simulink model "DealPosLrnd"  (R2018b)
settings: Solver=FixedStepDiscrete  StartTime=0.0  StopTime=10.0  FixedStep=0.01  RelTol=1e-3
undefined symbols (not defined in the file or in its folder): IfKeSMSbSeatMovBkRclnEnable_Val, IfKeSMSbSeatMovBlstOtwdInwdEnable_Val, IfKeSMSbSeatMovCshnFldEnable_Val, IfKeSMSbSeatMovCushnFrtEnable_Val, IfKeSMSbSeatMovFrwdBkwdEnable_Val, IfKeSMSbSeatMovFtrstEnable_Val, IfKeSMSbSeatMovLgrstEnable_Val, IfKeSMSbSeatMovLtwdRtwdEnable_Val, IfVeSMSeStNumConfig, KeSMSbArmscreenMovEnable_Val, KeSMSbIgnorePosLrnd_Val, KeSMSbSeatMovHdFrwdBkwdEnable_Val, KeSMSbSeatMovHdUpwdDnwdEnable_Val, KeSMSbSeatMovLgrstExpdEnable_Val
(part 1 of 2)
settings Model: Creator=su3dcu  LastModifiedBy=su3dcu
settings DataIOCC: SaveFormat=StructureWithTime  ReturnWorkspaceOutputs=on
settings OptimizationCC: DefaultParameterBehavior=Inlined  EnhancedBackFolding=on  PassReuseOutputArgsAs=Individual arguments  ZeroExternalMemoryAtStartup=off  ZeroInternalMemoryAtStartup=off  OptimizeBlockOrder=speed  DifferentSizesBufferReuse=on  OptimizationCustomize=off
settings DebuggingCC: ParameterTunabilityLossMsg=error
settings HardwareCC: ProdBitPerPointer=32  ProdBitPerSizeT=32  ProdBitPerPtrDiffT=32  ProdLargestAtomicFloat=None  ProdWordSize=32  ProdHWDeviceType=Renesas->RH850
settings ModelReferenceCC: ModelReferenceNumInstancesAllowed=Single
settings SFSimCC: SimCustomHeaderCode="#include\"Rte_Type.h\""  MATLABDynamicMemAlloc=off
settings RTWCC: SystemTargetFile=autosar.tlc  GenCodeOnly=on  TemplateMakefile=ert_default_tmf  Description=AUTOSAR  GenerateReport=on  IncludeHyperlinkInReport=on  LaunchReport=on  CodeExecutionProfiling=on  GenerateTraceInfo=on  GenerateTraceReport=on  GenerateTraceReportSl=on  GenerateTraceReportSf=on  GenerateTraceReportEml=on  GenerateCodeMetricsReport=on
settings CodeAppCC: ForceParamTrailComments=on  IgnoreCustomStorageClasses=off  MaxIdLength=63  OperatorAnnotations=on  SimulinkDataObjDesc=on  SFDataObjDesc=on  InsertBlockDesc=on
settings STFCustomTargetCC: TargetLangStandard=C99 (ISO)  MultiwordLength=256  ParMdlRefBuildCompliant=on  CompOptLevelCompliant=on  IncludeMdlTerminateFcn=off  CombineOutputUpdateFcns=on  SuppressErrorStatus=on  ERTCustomFileBanners=on  SupportAbsoluteTime=off  PurelyIntegerCode=on  SupportNonFinite=off  SupportComplex=off  SupportContinuousTime=off  SupportNonInlinedSFcns=off  RemoveResetFunc=on  MATLABClassNameForMDSCustomization=Simulink.SoftwareTarget.ERTCustomization  AutosarCompliant=on  UseToolchainInfoCompliant=on  LookupTableObjectStructAxisOrder=2,1,3,4,...  LUTObjectStructOrderEvenSpacing=Size,Table,Breakpoints  SystemTargetFile=autosar.tlc
settings ERTTargetCC: TargetLangStandard=C99 (ISO)  ConcurrentExecutionCompliant=off  IncludeMdlTerminateFcn=off  SuppressErrorStatus=on  SupportAbsoluteTime=off  PurelyIntegerCode=on  SupportNonFinite=off  SupportComplex=off  ModelStepFunctionPrototypeControlCompliant=off  CPPClassGenCompliant=off  AutosarCompliant=on  LookupTableObjectStructAxisOrder=2,1,3,4,...  LUTObjectStructOrderEvenSpacing=Size,Table,Breakpoints  InlinedParameterPlacement=NonHierarchical  ERTCustomFileTemplate=example_file_process.tlc  ERTFilePackagingFormat=Compact
settings ConfigComp: DVTestSuiteOptimization=CombinedObjectives (Nonlinear Extended)  DVDetectActiveLogic=on  DVDetectOutOfBounds=on

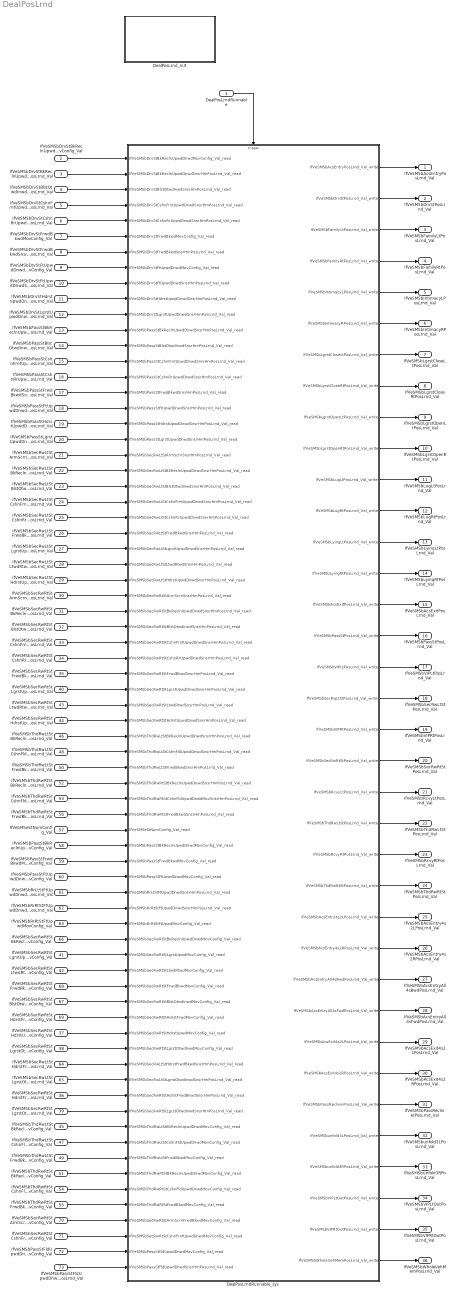
== system DealPosLrnd ==
  DealPosLrndRunnable : Inport  SampleTime=0.01  OutputFunctionCall=on
  IfVeSMSbDrvStBkReclnUpwdDnwdMovConfig_Val : Inport  Port=2  OutDataTypeStr=boolean  PortDimensions=1
  IfVeSMSbDrvStBkReclnUpwdDnwdSnsrHmPosLrnd_Val : Inport  Port=3  OutDataTypeStr=PosLrnd1  PortDimensions=1
  IfVeSMSbDrvStBlstOtwdInwdSnsrHmPosLrnd_Val : Inport  Port=4  OutDataTypeStr=PosLrnd1  PortDimensions=1
  IfVeSMSbDrvStCshnFrntUpwdDnwdSnsrHmPosLrnd_Val : Inport  Port=5  OutDataTypeStr=PosLrnd1  PortDimensions=1
  IfVeSMSbDrvStCshnRrUpwdDnwdSnsrHmPosLrnd_Val : Inport  Port=6  OutDataTypeStr=PosLrnd1  PortDimensions=1
  IfVeSMSbDrvStFrwdBkwdMovConfig_Val : Inport  Port=7  OutDataTypeStr=boolean  PortDimensions=1
  IfVeSMSbDrvStFrwdBkwdSnsrHmPosLrnd_Val : Inport  Port=8  OutDataTypeStr=PosLrnd1  PortDimensions=1
  IfVeSMSbDrvStFtUpwdDnwdMovConfig_Val : Inport  Port=9  OutDataTypeStr=boolean  PortDimensions=1
  IfVeSMSbDrvStFtUpwdDnwdSnsrHmPosLrnd_Val : Inport  Port=10  OutDataTypeStr=PosLrnd1  PortDimensions=1
  IfVeSMSbDrvStHdrstUpwdDnwdSnsrHmPosLrnd_Val : Inport  Port=11  OutDataTypeStr=PosLrnd1  PortDimensions=1
  IfVeSMSbDrvStLgrstUpwdDnwdSnsrHmPosLrnd_Val : Inport  Port=12  OutDataTypeStr=PosLrnd1  PortDimensions=1
  IfVeSMSbPassStBkReclnUpwdDnwdSnsrHmPosLrnd_Val : Inport  Port=13  OutDataTypeStr=PosLrnd1  PortDimensions=1
  IfVeSMSbPassStBlstOtwdInwdSnsrHmPosLrnd_Val : Inport  Port=14  OutDataTypeStr=PosLrnd1  PortDimensions=1
  IfVeSMSbPassStCshnFrntUpwdDnwdSnsrHmPosLrnd_Val : Inport  Port=15  OutDataTypeStr=PosLrnd1  PortDimensions=1
  IfVeSMSbPassStCshnRrUpwdDnwdSnsrHmPosLrnd_Val : Inport  Port=16  OutDataTypeStr=PosLrnd1  PortDimensions=1
  IfVeSMSbPassStFrwdBkwdSnsrHmPosLrnd_Val : Inport  Port=17  OutDataTypeStr=PosLrnd1  PortDimensions=1
  IfVeSMSbPassStFtUpwdDnwdSnsrHmPosLrnd_Val : Inport  Port=18  OutDataTypeStr=PosLrnd1  PortDimensions=1
  IfVeSMSbPassStHdrstUpwdDnwdSnsrHmPosLrnd_Val : Inport  Port=19  OutDataTypeStr=PosLrnd1  PortDimensions=1
  IfVeSMSbPassStLgrstUpwdDnwdSnsrHmPosLrnd_Val : Inport  Port=20  OutDataTypeStr=PosLrnd1  PortDimensions=1
  IfVeSMSbSecRwLtStArmScrnSnsrHmPosLrnd_Val : Inport  Port=21  OutDataTypeStr=PosLrnd1  PortDimensions=1
  IfVeSMSbSecRwLtStBkReclnUpwdDnwdSnsrHmPosLrnd_Val : Inport  Port=22  OutDataTypeStr=PosLrnd1  PortDimensions=1
  IfVeSMSbSecRwLtStBlstOtwdInwdSnsrHmPosLrnd_Val : Inport  Port=23  OutDataTypeStr=PosLrnd1  PortDimensions=1
  IfVeSMSbSecRwLtStCshnFrntUpwdDnwdSnsrHmPosLrnd_Val : Inport  Port=24  OutDataTypeStr=PosLrnd1  PortDimensions=1
  IfVeSMSbSecRwLtStCshnRrUpwdDnwdSnsrHmPosLrnd_Val : Inport  Port=25  OutDataTypeStr=PosLrnd1  PortDimensions=1
  IfVeSMSbSecRwLtStFrwdBkwdSnsrHmPosLrnd_Val : Inport  Port=26  OutDataTypeStr=PosLrnd1  PortDimensions=1
  IfVeSMSbSecRwLtStLgrstUpwdDnwdSnsrHmPosLrnd_Val : Inport  Port=27  OutDataTypeStr=PosLrnd1  PortDimensions=1
  IfVeSMSbSecRwLtStLtwdRtwdSnsrHmPosLrnd_Val : Inport  Port=28  OutDataTypeStr=PosLrnd1  PortDimensions=1
  IfVeSMSbSecRwLtStHdrstUpwdDnwdSnsrHmPosLrnd_Val : Inport  Port=29  OutDataTypeStr=PosLrnd1  PortDimensions=1
  IfVeSMSbSecRwRtStArmScrnSnsrHmPosLrnd_Val : Inport  Port=30  OutDataTypeStr=PosLrnd1  PortDimensions=1
  IfVeSMSbSecRwRtStBkReclnUpwdDnwdSnsrHmPosLrnd_Val : Inport  Port=31  OutDataTypeStr=PosLrnd1  PortDimensions=1
  IfVeSMSbSecRwRtStBlstOtwdInwdSnsrHmPosLrnd_Val : Inport  Port=32  OutDataTypeStr=PosLrnd1  PortDimensions=1
  IfVeSMSbSecRwRtStCshnFrntUpwdDnwdSnsrHmPosLrnd_Val : Inport  Port=33  OutDataTypeStr=PosLrnd1  PortDimensions=1
  IfVeSMSbSecRwRtStCshnRrUpwdDnwdSnsrHmPosLrnd_Val : Inport  Port=34  OutDataTypeStr=PosLrnd1  PortDimensions=1
  IfVeSMSbSecRwRtStFrwdBkwdSnsrHmPosLrnd_Val : Inport  Port=35  OutDataTypeStr=PosLrnd1  PortDimensions=1
  IfVeSMSbSecRwRtStHdrstFrwdBkwdSnsrHmPosLrnd_Val : Inport  Port=36  OutDataTypeStr=PosLrnd1  PortDimensions=1
  IfVeSMSbSecRwRtStHdrstUpwdMovConfig_Val : Inport  Port=37  OutDataTypeStr=boolean  PortDimensions=1
  IfVeSMSbSecRwRtStLgrstOtwdInwdMovConfig_Val : Inport  Port=38  OutDataTypeStr=boolean  PortDimensions=1
  IfVeSMSbSecRwRtStLgrstOtwdInwdSnsrHmPosLrnd_Val : Inport  Port=39  OutDataTypeStr=PosLrnd1  PortDimensions=1
  IfVeSMSbSecRwRtStLgrstUpwdDnwdSnsrHmPosLrnd_Val : Inport  Port=40  OutDataTypeStr=PosLrnd1  PortDimensions=1
  IfVeSMSbSecRwRtStLgrstUpwdMovConfig_Val : Inport  Port=41  OutDataTypeStr=boolean  PortDimensions=1
  IfVeSMSbSecRwRtStLtwdRtwdMovConfig_Val : Inport  Port=42  OutDataTypeStr=boolean  PortDimensions=1
  IfVeSMSbSecRwRtStLtwdRtwdSnsrHmPosLrnd_Val : Inport  Port=43  OutDataTypeStr=PosLrnd1  PortDimensions=1
  IfVeSMSbSecRwRtStHdrstUpwdDnwdSnsrHmPosLrnd_Val : Inport  Port=44  OutDataTypeStr=PosLrnd1  PortDimensions=1
  IfVeSMSbThdRwLtStBkReclnUpwdDnwdMovConfig_Val : Inport  Port=45  OutDataTypeStr=boolean  PortDimensions=1
  IfVeSMSbThdRwLtStBkReclnUpwdDnwdSnsrHmPosLrnd_Val : Inport  Port=46  OutDataTypeStr=PosLrnd1  PortDimensions=1
  IfVeSMSbThdRwLtStCshnFldUpwdDnwdMovConfig_Val : Inport  Port=47  OutDataTypeStr=boolean  PortDimensions=1
  IfVeSMSbThdRwLtStCshnFldUpwdDnwdSnsrHmPosLrnd_Val : Inport  Port=48  OutDataTypeStr=PosLrnd1  PortDimensions=1
  IfVeSMSbThdRwLtStFrwdBkwdMovConfig_Val : Inport  Port=49  OutDataTypeStr=boolean  PortDimensions=1
  IfVeSMSbThdRwLtStFrwdBkwdSnsrHmPosLrnd_Val : Inport  Port=50  OutDataTypeStr=PosLrnd1  PortDimensions=1
  IfVeSMSbThdRwRtStBkReclnUpwdDnwdMovConfig_Val : Inport  Port=51  OutDataTypeStr=boolean  PortDimensions=1
  IfVeSMSbThdRwRtStBkReclnUpwdDnwdSnsrHmPosLrnd_Val : Inport  Port=52  OutDataTypeStr=PosLrnd1  PortDimensions=1
  IfVeSMSbThdRwRtStCshnFldUpwdDnwdMovSnsrHmPosLrnd_Val : Inport  Port=53  OutDataTypeStr=PosLrnd1  PortDimensions=1
  IfVeSMSbThdRwRtStCshnFldUpwdDnwdMovConfig_Val : Inport  Port=54  OutDataTypeStr=boolean  PortDimensions=1
  IfVeSMSbThdRwRtStFrwdBkwdMovConfig_Val : Inport  Port=55  OutDataTypeStr=boolean  PortDimensions=1
  IfVeSMSbThdRwRtStFrwdBkwdSnsrHmPosLrnd_Val : Inport  Port=56  OutDataTypeStr=PosLrnd1  PortDimensions=1
  IfVeSMSeStNumConfig_Val : Inport  Port=57  OutDataTypeStr=Enum: IfVeSMSeStNumConfig  PortDimensions=1
  IfVeSMSbPassStBkReclnUpwdDnwdMovConfig_Val : Inport  Port=58  OutDataTypeStr=boolean  PortDimensions=1
  IfVeSMSbPassStFrwdBkwdMovConfig_Val : Inport  Port=59  OutDataTypeStr=boolean  PortDimensions=1
  IfVeSMSbPassStFtUpwdDnwdMovConfig_Val : Inport  Port=60  OutDataTypeStr=boolean  PortDimensions=1
  IfVeSMSbRrLtStFtUpwdDnwdSnsrHmPosLrnd_Val : Inport  Port=61  OutDataTypeStr=PosLrnd1  PortDimensions=1
  IfVeSMSbRrRtStFtUpwdDnwdSnsrHmPosLrnd_Val : Inport  Port=62  OutDataTypeStr=PosLrnd1  PortDimensions=1
  IfVeSMSbRrRtStFtUpwdMovConfig_Val : Inport  Port=63  OutDataTypeStr=boolean  PortDimensions=1
  IfVeSMSbSecRwLtStHdrstFrwdBkwdSnsrHmPosLrnd_Val : Inport  Port=64  OutDataTypeStr=PosLrnd1  PortDimensions=1
  IfVeSMSbSecRwLtStLgrstOtwdInwdSnsrHmPosLrnd_Val : Inport  Port=65  OutDataTypeStr=PosLrnd1  PortDimensions=1
  IfVeSMSbSecRwRtStBkReclnUpwdDnwdMovConfig_Val : Inport  Port=66  OutDataTypeStr=boolean  PortDimensions=1
  IfVeSMSbSecRwRtStBlstOtwdInwdMovConfig_Val : Inport  Port=67  OutDataTypeStr=boolean  PortDimensions=1
  IfVeSMSbSecRwRtStFrwdBkwdMovConfig_Val : Inport  Port=68  OutDataTypeStr=boolean  PortDimensions=1
  IfVeSMSbSecRwRtStHdrstFrwdMovConfig_Val : Inport  Port=69  OutDataTypeStr=boolean  PortDimensions=1
  IfVeSMSbSecRwRtStArmScrnFrwdBkwdMovConfig_Val : Inport  Port=70  OutDataTypeStr=boolean  PortDimensions=1
  IfVeSMSbSecRwRtStCshnFrntUpwdDnwdMovConfig_Val : Inport  Port=71  OutDataTypeStr=boolean  PortDimensions=1
  IfVeSMSbPassStFldUpwdDnwdMovConfig_Val : Inport  Port=72  OutDataTypeStr=boolean  PortDimensions=1
  IfVeSMSbPassStFldUpwdDnwdSnsrHmPosLrnd_Val : Inport  Port=73  OutDataTypeStr=PosLrnd1  PortDimensions=1
  DealPosLrndRunnable_sys : Subsystem
  DealPosLrnd_Init : Subsystem
  IfVeSMSbAcsEntryPosLrnd_Val : Outport  OutDataTypeStr=PosLrnd1  PortDimensions=1
  IfVeSMSbDrvStPosLrnd_Val : Outport  Port=2  OutDataTypeStr=PosLrnd1  PortDimensions=1
  IfVeSMSbFamilyLtPosLrnd_Val : Outport  Port=3  OutDataTypeStr=PosLrnd1  PortDimensions=1
  IfVeSMSbFamilyRtPosLrnd_Val : Outport  Port=4  OutDataTypeStr=PosLrnd1  PortDimensions=1
  IfVeSMSbIntimacyLPosLrnd_Val : Outport  Port=5  OutDataTypeStr=PosLrnd1  PortDimensions=1
  IfVeSMSbIntimacyRPosLrnd_Val : Outport  Port=6  OutDataTypeStr=PosLrnd1  PortDimensions=1
  IfVeSMSbLgrstCloseLtPosLrnd_Val : Outport  Port=7  OutDataTypeStr=PosLrnd1  PortDimensions=1
  IfVeSMSbLgrstCloseRtPosLrnd_Val : Outport  Port=8  OutDataTypeStr=PosLrnd1  PortDimensions=1
  IfVeSMSbLgrstOpenLtPosLrnd_Val : Outport  Port=9  OutDataTypeStr=PosLrnd1  PortDimensions=1
  IfVeSMSbLgrstOpenRtPosLrnd_Val : Outport  Port=10  OutDataTypeStr=PosLrnd1  PortDimensions=1
  IfVeSMSbLugLtPosLrnd_Val : Outport  Port=11  OutDataTypeStr=PosLrnd1  PortDimensions=1
  IfVeSMSbLugRtPosLrnd_Val : Outport  Port=12  OutDataTypeStr=PosLrnd1  PortDimensions=1
  IfVeSMSbLyingLtPosLrnd_Val : Outport  Port=13  OutDataTypeStr=PosLrnd1  PortDimensions=1
  IfVeSMSbLyingRtPosLrnd_Val : Outport  Port=14  OutDataTypeStr=PosLrnd1  PortDimensions=1
  IfVeSMSbAcsExitPosLrnd_Val : Outport  Port=15  OutDataTypeStr=PosLrnd1  PortDimensions=1
  IfVeSMSbPassStPosLrnd_Val : Outport  Port=16  OutDataTypeStr=PosLrnd1  PortDimensions=1
  IfVeSMSbVIPLtPosLrnd_Val : Outport  Port=17  OutDataTypeStr=PosLrnd1  PortDimensions=1
  IfVeSMSbSecRwLtStPosLrnd_Val : Outport  Port=18  OutDataTypeStr=PosLrnd1  PortDimensions=1
  IfVeSMSbVIPRtPosLrnd_Val : Outport  Port=19  OutDataTypeStr=PosLrnd1  PortDimensions=1
  IfVeSMSbSecRwRtStPosLrnd_Val : Outport  Port=20  OutDataTypeStr=PosLrnd1  PortDimensions=1
  IfVeSMSbRcvyLtPosLrnd_Val : Outport  Port=21  OutDataTypeStr=PosLrnd1  PortDimensions=1
  IfVeSMSbThdRwLtStPosLrnd_Val : Outport  Port=22  OutDataTypeStr=PosLrnd1  PortDimensions=1
  IfVeSMSbRcvyRtPosLrnd_Val : Outport  Port=23  OutDataTypeStr=PosLrnd1  PortDimensions=1
  IfVeSMSbThdRwRtStPosLrnd_Val : Outport  Port=24  OutDataTypeStr=PosLrnd1  PortDimensions=1
  IfVeSMSbAcsEntry4s2LPosLrnd_Val : Outport  Port=25  OutDataTypeStr=PosLrnd1  PortDimensions=1
  IfVeSMSbAcsEntry4s2RPosLrnd_Val : Outport  Port=26  OutDataTypeStr=PosLrnd1  PortDimensions=1
  IfVeSMSbAcsEntryAll4sBwdPosLrnd_Val : Outport  Port=27  OutDataTypeStr=PosLrnd1  PortDimensions=1
  IfVeSMSbAcsEntryAll4sFwdPosLrnd_Val : Outport  Port=28  OutDataTypeStr=PosLrnd1  PortDimensions=1
  IfVeSMSbAcsExit4s2LPosLrnd_Val : Outport  Port=29  OutDataTypeStr=PosLrnd1  PortDimensions=1
  IfVeSMSbAcsExit4s2RPosLrnd_Val : Outport  Port=30  OutDataTypeStr=PosLrnd1  PortDimensions=1
  IfVeSMSbPassReclinerPosLrnd_Val : Outport  Port=31  OutDataTypeStr=PosLrnd1  PortDimensions=1
  IfVeSMSbunfold3LPosLrnd_Val : Outport  Port=32  OutDataTypeStr=PosLrnd1  PortDimensions=1
  IfVeSMSbunfold3RPosLrnd_Val : Outport  Port=33  OutDataTypeStr=PosLrnd1  PortDimensions=1
  IfVeSMSbVIPLtOutPosLrnd_Val : Outport  Port=34  OutDataTypeStr=PosLrnd1  PortDimensions=1
  IfVeSMSbVIPRtOutPosLrnd_Val : Outport  Port=35  OutDataTypeStr=PosLrnd1  PortDimensions=1
  IfVeSMSbWholeVehMemPosLrnd_Val : Outport  Port=36  OutDataTypeStr=PosLrnd1  PortDimensions=1
  wires:
  IfVeSMSbDrvStBkReclnUpwdDnwdMovConfig_Val/1 -> DealPosLrndRunnable_sys/1(IfVeSMSbDrvStBkReclnUpwdDnwdMovConfig_Val_read)
  IfVeSMSbDrvStBkReclnUpwdDnwdSnsrHmPosLrnd_Val/1 -> DealPosLrndRunnable_sys/2(IfVeSMSbDrvStBkReclnUpwdDnwdSnsrHmPosLrnd_Val_read)
  IfVeSMSbDrvStBlstOtwdInwdSnsrHmPosLrnd_Val/1 -> DealPosLrndRunnable_sys/3(IfVeSMSbDrvStBlstOtwdInwdSnsrHmPosLrnd_Val_read)
  IfVeSMSbDrvStCshnFrntUpwdDnwdSnsrHmPosLrnd_Val/1 -> DealPosLrndRunnable_sys/4(IfVeSMSbDrvStCshnFrntUpwdDnwdSnsrHmPosLrnd_Val_read)
  IfVeSMSbDrvStCshnRrUpwdDnwdSnsrHmPosLrnd_Val/1 -> DealPosLrndRunnable_sys/5(IfVeSMSbDrvStCshnRrUpwdDnwdSnsrHmPosLrnd_Val_read)
  IfVeSMSbDrvStFrwdBkwdMovConfig_Val/1 -> DealPosLrndRunnable_sys/6(IfVeSMSbDrvStFrwdBkwdMovConfig_Val_read)
  IfVeSMSbDrvStFrwdBkwdSnsrHmPosLrnd_Val/1 -> DealPosLrndRunnable_sys/7(IfVeSMSbDrvStFrwdBkwdSnsrHmPosLrnd_Val_read)
  IfVeSMSbDrvStFtUpwdDnwdMovConfig_Val/1 -> DealPosLrndRunnable_sys/8(IfVeSMSbDrvStFtUpwdDnwdMovConfig_Val_read)
  IfVeSMSbDrvStFtUpwdDnwdSnsrHmPosLrnd_Val/1 -> DealPosLrndRunnable_sys/9(IfVeSMSbDrvStFtUpwdDnwdSnsrHmPosLrnd_Val_read)
  IfVeSMSbDrvStHdrstUpwdDnwdSnsrHmPosLrnd_Val/1 -> DealPosLrndRunnable_sys/10(IfVeSMSbDrvStHdrstUpwdDnwdSnsrHmPosLrnd_Val_read)
  IfVeSMSbDrvStLgrstUpwdDnwdSnsrHmPosLrnd_Val/1 -> DealPosLrndRunnable_sys/11(IfVeSMSbDrvStLgrstUpwdDnwdSnsrHmPosLrnd_Val_read)
  IfVeSMSbPassStBkReclnUpwdDnwdSnsrHmPosLrnd_Val/1 -> DealPosLrndRunnable_sys/12(IfVeSMSbPassStBkReclnUpwdDnwdSnsrHmPosLrnd_Val_read)
  IfVeSMSbPassStBlstOtwdInwdSnsrHmPosLrnd_Val/1 -> DealPosLrndRunnable_sys/13(IfVeSMSbPassStBlstOtwdInwdSnsrHmPosLrnd_Val_read)
  IfVeSMSbPassStCshnFrntUpwdDnwdSnsrHmPosLrnd_Val/1 -> DealPosLrndRunnable_sys/14(IfVeSMSbPassStCshnFrntUpwdDnwdSnsrHmPosLrnd_Val_read)
  IfVeSMSbPassStCshnRrUpwdDnwdSnsrHmPosLrnd_Val/1 -> DealPosLrndRunnable_sys/15(IfVeSMSbPassStCshnRrUpwdDnwdSnsrHmPosLrnd_Val_read)
  IfVeSMSbPassStFrwdBkwdSnsrHmPosLrnd_Val/1 -> DealPosLrndRunnable_sys/16(IfVeSMSbPassStFrwdBkwdSnsrHmPosLrnd_Val_read)
  IfVeSMSbPassStFtUpwdDnwdSnsrHmPosLrnd_Val/1 -> DealPosLrndRunnable_sys/17(IfVeSMSbPassStFtUpwdDnwdSnsrHmPosLrnd_Val_read)
  IfVeSMSbPassStHdrstUpwdDnwdSnsrHmPosLrnd_Val/1 -> DealPosLrndRunnable_sys/18(IfVeSMSbPassStHdrstUpwdDnwdSnsrHmPosLrnd_Val_read)
  IfVeSMSbPassStLgrstUpwdDnwdSnsrHmPosLrnd_Val/1 -> DealPosLrndRunnable_sys/19(IfVeSMSbPassStLgrstUpwdDnwdSnsrHmPosLrnd_Val_read)
  IfVeSMSbSecRwLtStArmScrnSnsrHmPosLrnd_Val/1 -> DealPosLrndRunnable_sys/20(IfVeSMSbSecRwLtStArmScrnSnsrHmPosLrnd_Val_read)
  IfVeSMSbSecRwLtStBkReclnUpwdDnwdSnsrHmPosLrnd_Val/1 -> DealPosLrndRunnable_sys/21(IfVeSMSbSecRwLtStBkReclnUpwdDnwdSnsrHmPosLrnd_Val_read)
  IfVeSMSbSecRwLtStBlstOtwdInwdSnsrHmPosLrnd_Val/1 -> DealPosLrndRunnable_sys/22(IfVeSMSbSecRwLtStBlstOtwdInwdSnsrHmPosLrnd_Val_read)
  IfVeSMSbSecRwLtStCshnFrntUpwdDnwdSnsrHmPosLrnd_Val/1 -> DealPosLrndRunnable_sys/23(IfVeSMSbSecRwLtStCshnFrntUpwdDnwdSnsrHmPosLrnd_Val_read)
  IfVeSMSbSecRwLtStCshnRrUpwdDnwdSnsrHmPosLrnd_Val/1 -> DealPosLrndRunnable_sys/24(IfVeSMSbSecRwLtStCshnRrUpwdDnwdSnsrHmPosLrnd_Val_read)
  IfVeSMSbSecRwLtStFrwdBkwdSnsrHmPosLrnd_Val/1 -> DealPosLrndRunnable_sys/25(IfVeSMSbSecRwLtStFrwdBkwdSnsrHmPosLrnd_Val_read)
  IfVeSMSbSecRwLtStLgrstUpwdDnwdSnsrHmPosLrnd_Val/1 -> DealPosLrndRunnable_sys/26(IfVeSMSbSecRwLtStLgrstUpwdDnwdSnsrHmPosLrnd_Val_read)
  IfVeSMSbSecRwLtStLtwdRtwdSnsrHmPosLrnd_Val/1 -> DealPosLrndRunnable_sys/27(IfVeSMSbSecRwLtStLtwdRtwdSnsrHmPosLrnd_Val_read)
  IfVeSMSbSecRwLtStHdrstUpwdDnwdSnsrHmPosLrnd_Val/1 -> DealPosLrndRunnable_sys/28(IfVeSMSbSecRwLtStHdrstUpwdDnwdSnsrHmPosLrnd_Val_read)
  IfVeSMSbSecRwRtStArmScrnSnsrHmPosLrnd_Val/1 -> DealPosLrndRunnable_sys/29(IfVeSMSbSecRwRtStArmScrnSnsrHmPosLrnd_Val_read)
  IfVeSMSbSecRwRtStBkReclnUpwdDnwdSnsrHmPosLrnd_Val/1 -> DealPosLrndRunnable_sys/30(IfVeSMSbSecRwRtStBkReclnUpwdDnwdSnsrHmPosLrnd_Val_read)
  IfVeSMSbSecRwRtStBlstOtwdInwdSnsrHmPosLrnd_Val/1 -> DealPosLrndRunnable_sys/31(IfVeSMSbSecRwRtStBlstOtwdInwdSnsrHmPosLrnd_Val_read)
  IfVeSMSbSecRwRtStCshnFrntUpwdDnwdSnsrHmPosLrnd_Val/1 -> DealPosLrndRunnable_sys/32(IfVeSMSbSecRwRtStCshnFrntUpwdDnwdSnsrHmPosLrnd_Val_read)
  IfVeSMSbSecRwRtStCshnRrUpwdDnwdSnsrHmPosLrnd_Val/1 -> DealPosLrndRunnable_sys/33(IfVeSMSbSecRwRtStCshnRrUpwdDnwdSnsrHmPosLrnd_Val_read)
  IfVeSMSbSecRwRtStFrwdBkwdSnsrHmPosLrnd_Val/1 -> DealPosLrndRunnable_sys/34(IfVeSMSbSecRwRtStFrwdBkwdSnsrHmPosLrnd_Val_read)
  IfVeSMSbSecRwRtStLgrstUpwdDnwdSnsrHmPosLrnd_Val/1 -> DealPosLrndRunnable_sys/35(IfVeSMSbSecRwRtStLgrstUpwdDnwdSnsrHmPosLrnd_Val_read)
  IfVeSMSbSecRwRtStLtwdRtwdSnsrHmPosLrnd_Val/1 -> DealPosLrndRunnable_sys/36(IfVeSMSbSecRwRtStLtwdRtwdSnsrHmPosLrnd_Val_read)
  IfVeSMSbSecRwRtStHdrstUpwdDnwdSnsrHmPosLrnd_Val/1 -> DealPosLrndRunnable_sys/37(IfVeSMSbSecRwRtStHdrstUpwdDnwdSnsrHmPosLrnd_Val_read)
  IfVeSMSbThdRwLtStBkReclnUpwdDnwdSnsrHmPosLrnd_Val/1 -> DealPosLrndRunnable_sys/38(IfVeSMSbThdRwLtStBkReclnUpwdDnwdSnsrHmPosLrnd_Val_read)
  IfVeSMSbThdRwLtStCshnFldUpwdDnwdSnsrHmPosLrnd_Val/1 -> DealPosLrndRunnable_sys/39(IfVeSMSbThdRwLtStCshnFldUpwdDnwdSnsrHmPosLrnd_Val_read)
  IfVeSMSbThdRwLtStFrwdBkwdSnsrHmPosLrnd_Val/1 -> DealPosLrndRunnable_sys/40(IfVeSMSbThdRwLtStFrwdBkwdSnsrHmPosLrnd_Val_read)
  IfVeSMSbThdRwRtStBkReclnUpwdDnwdSnsrHmPosLrnd_Val/1 -> DealPosLrndRunnable_sys/41(IfVeSMSbThdRwRtStBkReclnUpwdDnwdSnsrHmPosLrnd_Val_read)
  IfVeSMSbThdRwRtStCshnFldUpwdDnwdMovSnsrHmPosLrnd_Val/1 -> DealPosLrndRunnable_sys/42(IfVeSMSbThdRwRtStCshnFldUpwdDnwdMovSnsrHmPosLrnd_Val_read)
  IfVeSMSbThdRwRtStFrwdBkwdSnsrHmPosLrnd_Val/1 -> DealPosLrndRunnable_sys/43(IfVeSMSbThdRwRtStFrwdBkwdSnsrHmPosLrnd_Val_read)
  IfVeSMSeStNumConfig_Val/1 -> DealPosLrndRunnable_sys/44(IfVeSMSeStNumConfig_Val_read)
  DealPosLrndRunnable_sys/1(IfVeSMSbAcsEntryPosLrnd_Val_write) -> IfVeSMSbAcsEntryPosLrnd_Val/1
  DealPosLrndRunnable_sys/2(IfVeSMSbDrvStPosLrnd_Val_write) -> IfVeSMSbDrvStPosLrnd_Val/1
  DealPosLrndRunnable_sys/3(IfVeSMSbFamilyLtPosLrnd_Val_write) -> IfVeSMSbFamilyLtPosLrnd_Val/1
  DealPosLrndRunnable_sys/4(IfVeSMSbFamilyRtPosLrnd_Val_write) -> IfVeSMSbFamilyRtPosLrnd_Val/1
  DealPosLrndRunnable_sys/5(IfVeSMSbIntimacyLPosLrnd_Val_write) -> IfVeSMSbIntimacyLPosLrnd_Val/1
  DealPosLrndRunnable_sys/6(IfVeSMSbIntimacyRPosLrnd_Val_write) -> IfVeSMSbIntimacyRPosLrnd_Val/1
  DealPosLrndRunnable_sys/7(IfVeSMSbLgrstCloseLtPosLrnd_Val_write) -> IfVeSMSbLgrstCloseLtPosLrnd_Val/1
  DealPosLrndRunnable_sys/8(IfVeSMSbLgrstCloseRtPosLrnd_Val_write) -> IfVeSMSbLgrstCloseRtPosLrnd_Val/1
  DealPosLrndRunnable_sys/9(IfVeSMSbLgrstOpenLtPosLrnd_Val_write) -> IfVeSMSbLgrstOpenLtPosLrnd_Val/1
  DealPosLrndRunnable_sys/10(IfVeSMSbLgrstOpenRtPosLrnd_Val_write) -> IfVeSMSbLgrstOpenRtPosLrnd_Val/1
  DealPosLrndRunnable_sys/11(IfVeSMSbLugLtPosLrnd_Val_write) -> IfVeSMSbLugLtPosLrnd_Val/1
  DealPosLrndRunnable_sys/12(IfVeSMSbLugRtPosLrnd_Val_write) -> IfVeSMSbLugRtPosLrnd_Val/1
  DealPosLrndRunnable_sys/13(IfVeSMSbLyingLtPosLrnd_Val_write) -> IfVeSMSbLyingLtPosLrnd_Val/1
  DealPosLrndRunnable_sys/14(IfVeSMSbLyingRtPosLrnd_Val_write) -> IfVeSMSbLyingRtPosLrnd_Val/1
  DealPosLrndRunnable_sys/15(IfVeSMSbAcsExitPosLrnd_Val_write) -> IfVeSMSbAcsExitPosLrnd_Val/1
  DealPosLrndRunnable_sys/16(IfVeSMSbPassStPosLrnd_Val_write) -> IfVeSMSbPassStPosLrnd_Val/1
  DealPosLrndRunnable_sys/17(IfVeSMSbVIPLtPosLrnd_Val_write) -> IfVeSMSbVIPLtPosLrnd_Val/1
  DealPosLrndRunnable_sys/18(IfVeSMSbSecRwLtStPosLrnd_Val_write) -> IfVeSMSbSecRwLtStPosLrnd_Val/1
  DealPosLrndRunnable_sys/19(IfVeSMSbVIPRtPosLrnd_Val_write) -> IfVeSMSbVIPRtPosLrnd_Val/1
  DealPosLrndRunnable_sys/20(IfVeSMSbSecRwRtStPosLrnd_Val_write) -> IfVeSMSbSecRwRtStPosLrnd_Val/1
  DealPosLrndRunnable_sys/21(IfVeSMSbRcvyLtPosLrnd_Val_write) -> IfVeSMSbRcvyLtPosLrnd_Val/1
  DealPosLrndRunnable_sys/22(IfVeSMSbThdRwLtStPosLrnd_Val_write) -> IfVeSMSbThdRwLtStPosLrnd_Val/1
  DealPosLrndRunnable_sys/23(IfVeSMSbRcvyRtPosLrnd_Val_write) -> IfVeSMSbRcvyRtPosLrnd_Val/1
  DealPosLrndRunnable_sys/24(IfVeSMSbThdRwRtStPosLrnd_Val_write) -> IfVeSMSbThdRwRtStPosLrnd_Val/1
  DealPosLrndRunnable/1 -> DealPosLrndRunnable_sys/Trigger
  IfVeSMSbPassStBkReclnUpwdDnwdMovConfig_Val/1 -> DealPosLrndRunnable_sys/45(IfVeSMSbPassStBkReclnUpwdDnwdMovConfig_Val_read)
  IfVeSMSbPassStFrwdBkwdMovConfig_Val/1 -> DealPosLrndRunnable_sys/46(IfVeSMSbPassStFrwdBkwdMovConfig_Val_read)
  IfVeSMSbPassStFtUpwdDnwdMovConfig_Val/1 -> DealPosLrndRunnable_sys/47(IfVeSMSbPassStFtUpwdDnwdMovConfig_Val_read)
  IfVeSMSbRrLtStFtUpwdDnwdSnsrHmPosLrnd_Val/1 -> DealPosLrndRunnable_sys/48(IfVeSMSbRrLtStFtUpwdDnwdSnsrHmPosLrnd_Val_read)
  IfVeSMSbRrRtStFtUpwdDnwdSnsrHmPosLrnd_Val/1 -> DealPosLrndRunnable_sys/49(IfVeSMSbRrRtStFtUpwdDnwdSnsrHmPosLrnd_Val_read)
  IfVeSMSbRrRtStFtUpwdMovConfig_Val/1 -> DealPosLrndRunnable_sys/50(IfVeSMSbRrRtStFtUpwdMovConfig_Val_read)
  IfVeSMSbSecRwRtStBkReclnUpwdDnwdMovConfig_Val/1 -> DealPosLrndRunnable_sys/51(IfVeSMSbSecRwRtStBkReclnUpwdDnwdMovConfig_Val_read)
  IfVeSMSbSecRwLtStHdrstFrwdBkwdSnsrHmPosLrnd_Val/1 -> DealPosLrndRunnable_sys/59(IfVeSMSbSecRwLtStHdrstFrwdBkwdSnsrHmPosLrnd_Val_read)
  IfVeSMSbSecRwLtStLgrstOtwdInwdSnsrHmPosLrnd_Val/1 -> DealPosLrndRunnable_sys/60(IfVeSMSbSecRwLtStLgrstOtwdInwdSnsrHmPosLrnd_Val_read)
  IfVeSMSbSecRwRtStBlstOtwdInwdMovConfig_Val/1 -> DealPosLrndRunnable_sys/55(IfVeSMSbSecRwRtStBlstOtwdInwdMovConfig_Val_read)
  IfVeSMSbSecRwRtStFrwdBkwdMovConfig_Val/1 -> DealPosLrndRunnable_sys/54(IfVeSMSbSecRwRtStFrwdBkwdMovConfig_Val_read)
  IfVeSMSbSecRwRtStHdrstFrwdMovConfig_Val/1 -> DealPosLrndRunnable_sys/56(IfVeSMSbSecRwRtStHdrstFrwdMovConfig_Val_read)
  IfVeSMSbSecRwRtStLgrstUpwdMovConfig_Val/1 -> DealPosLrndRunnable_sys/52(IfVeSMSbSecRwRtStLgrstUpwdMovConfig_Val_read)
  IfVeSMSbSecRwRtStLtwdRtwdMovConfig_Val/1 -> DealPosLrndRunnable_sys/53(IfVeSMSbSecRwRtStLtwdRtwdMovConfig_Val_read)
  IfVeSMSbSecRwRtStHdrstUpwdMovConfig_Val/1 -> DealPosLrndRunnable_sys/57(IfVeSMSbSecRwRtStHdrstUpwdMovConfig_Val_read)
  IfVeSMSbSecRwRtStLgrstOtwdInwdMovConfig_Val/1 -> DealPosLrndRunnable_sys/58(IfVeSMSbSecRwRtStLgrstOtwdInwdMovConfig_Val_read)
  IfVeSMSbSecRwRtStLgrstOtwdInwdSnsrHmPosLrnd_Val/1 -> DealPosLrndRunnable_sys/62(IfVeSMSbSecRwRtStLgrstOtwdInwdSnsrHmPosLrnd_Val_read)
  IfVeSMSbSecRwRtStHdrstFrwdBkwdSnsrHmPosLrnd_Val/1 -> DealPosLrndRunnable_sys/61(IfVeSMSbSecRwRtStHdrstFrwdBkwdSnsrHmPosLrnd_Val_read)
  IfVeSMSbThdRwLtStBkReclnUpwdDnwdMovConfig_Val/1 -> DealPosLrndRunnable_sys/63(IfVeSMSbThdRwLtStBkReclnUpwdDnwdMovConfig_Val_read)
  IfVeSMSbThdRwLtStCshnFldUpwdDnwdMovConfig_Val/1 -> DealPosLrndRunnable_sys/64(IfVeSMSbThdRwLtStCshnFldUpwdDnwdMovConfig_Val_read)
  IfVeSMSbThdRwLtStFrwdBkwdMovConfig_Val/1 -> DealPosLrndRunnable_sys/65(IfVeSMSbThdRwLtStFrwdBkwdMovConfig_Val_read)
  IfVeSMSbThdRwRtStBkReclnUpwdDnwdMovConfig_Val/1 -> DealPosLrndRunnable_sys/66(IfVeSMSbThdRwRtStBkReclnUpwdDnwdMovConfig_Val_read)
  IfVeSMSbThdRwRtStCshnFldUpwdDnwdMovConfig_Val/1 -> DealPosLrndRunnable_sys/67(IfVeSMSbThdRwRtStCshnFldUpwdDnwdMovConfig_Val_read)
  IfVeSMSbThdRwRtStFrwdBkwdMovConfig_Val/1 -> DealPosLrndRunnable_sys/68(IfVeSMSbThdRwRtStFrwdBkwdMovConfig_Val_read)
  DealPosLrndRunnable_sys/25(IfVeSMSbAcsEntry4s2LPosLrnd_Val_write) -> IfVeSMSbAcsEntry4s2LPosLrnd_Val/1
  DealPosLrndRunnable_sys/26(IfVeSMSbAcsEntry4s2RPosLrnd_Val_write) -> IfVeSMSbAcsEntry4s2RPosLrnd_Val/1
  DealPosLrndRunnable_sys/27(IfVeSMSbAcsEntryAll4sBwdPosLrnd_Val_write) -> IfVeSMSbAcsEntryAll4sBwdPosLrnd_Val/1
  DealPosLrndRunnable_sys/28(IfVeSMSbAcsEntryAll4sFwdPosLrnd_Val_write) -> IfVeSMSbAcsEntryAll4sFwdPosLrnd_Val/1
  DealPosLrndRunnable_sys/29(IfVeSMSbAcsExit4s2LPosLrnd_Val_write) -> IfVeSMSbAcsExit4s2LPosLrnd_Val/1
  DealPosLrndRunnable_sys/30(IfVeSMSbAcsExit4s2RPosLrnd_Val_write) -> IfVeSMSbAcsExit4s2RPosLrnd_Val/1
  IfVeSMSbSecRwRtStArmScrnFrwdBkwdMovConfig_Val/1 -> DealPosLrndRunnable_sys/69(IfVeSMSbSecRwRtStArmScrnFrwdBkwdMovConfig_Val_read)
  IfVeSMSbSecRwRtStCshnFrntUpwdDnwdMovConfig_Val/1 -> DealPosLrndRunnable_sys/70(IfVeSMSbSecRwRtStCshnFrntUpwdDnwdMovConfig_Val_read)
  IfVeSMSbPassStFldUpwdDnwdMovConfig_Val/1 -> DealPosLrndRunnable_sys/71(IfVeSMSbPassStFldUpwdDnwdMovConfig_Val_read)
  IfVeSMSbPassStFldUpwdDnwdSnsrHmPosLrnd_Val/1 -> DealPosLrndRunnable_sys/72(IfVeSMSbPassStFldUpwdDnwdSnsrHmPosLrnd_Val_read)
  DealPosLrndRunnable_sys/31(IfVeSMSbPassReclinerPosLrnd_Val_write) -> IfVeSMSbPassReclinerPosLrnd_Val/1
  DealPosLrndRunnable_sys/32(IfVeSMSbunfold3LPosLrnd_Val_write) -> IfVeSMSbunfold3LPosLrnd_Val/1
  DealPosLrndRunnable_sys/33(IfVeSMSbunfold3RPosLrnd_Val_write) -> IfVeSMSbunfold3RPosLrnd_Val/1
  DealPosLrndRunnable_sys/34(IfVeSMSbVIPLtOutPosLrnd_Val_write) -> IfVeSMSbVIPLtOutPosLrnd_Val/1
  DealPosLrndRunnable_sys/35(IfVeSMSbVIPRtOutPosLrnd_Val_write) -> IfVeSMSbVIPRtOutPosLrnd_Val/1
  DealPosLrndRunnable_sys/36(IfVeSMSbWholeVehMemPosLrnd_Val_write) -> IfVeSMSbWholeVehMemPosLrnd_Val/1

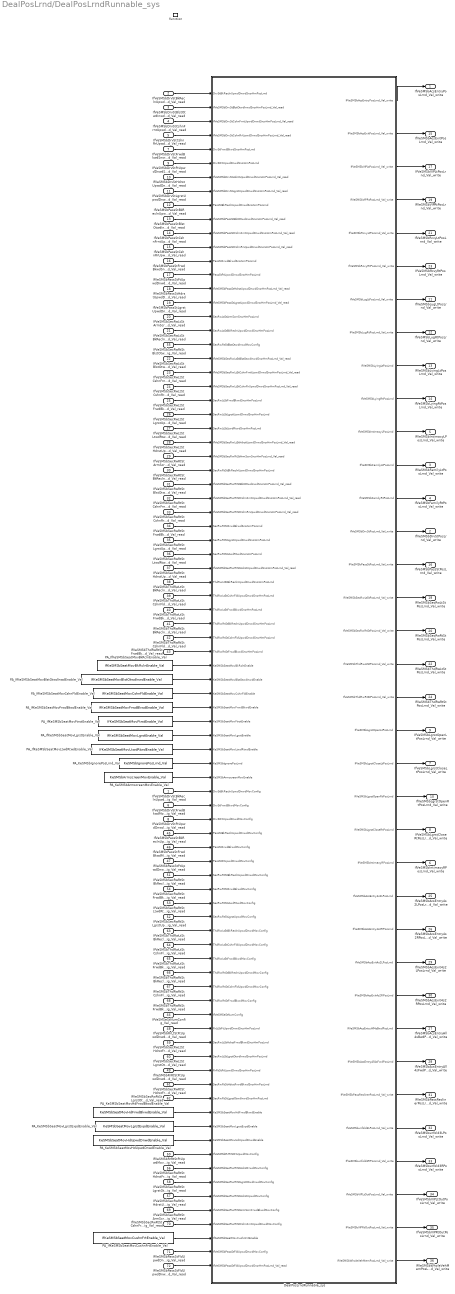
== system DealPosLrnd/DealPosLrndRunnable_sys ==
  IfVeSMSbDrvStBkReclnUpwdDnwdMovConfig_Val_read : Inport
  IfVeSMSbDrvStBkReclnUpwdDnwdSnsrHmPosLrnd_Val_read : Inport  Port=2
  IfVeSMSbDrvStBlstOtwdInwdSnsrHmPosLrnd_Val_read : Inport  Port=3
  IfVeSMSbDrvStCshnFrntUpwdDnwdSnsrHmPosLrnd_Val_read : Inport  Port=4
  IfVeSMSbDrvStCshnRrUpwdDnwdSnsrHmPosLrnd_Val_read : Inport  Port=5
  IfVeSMSbDrvStFrwdBkwdMovConfig_Val_read : Inport  Port=6
  IfVeSMSbDrvStFrwdBkwdSnsrHmPosLrnd_Val_read : Inport  Port=7
  IfVeSMSbDrvStFtUpwdDnwdMovConfig_Val_read : Inport  Port=8
  IfVeSMSbDrvStFtUpwdDnwdSnsrHmPosLrnd_Val_read : Inport  Port=9
  IfVeSMSbDrvStHdrstUpwdDnwdSnsrHmPosLrnd_Val_read : Inport  Port=10
  IfVeSMSbDrvStLgrstUpwdDnwdSnsrHmPosLrnd_Val_read : Inport  Port=11
  IfVeSMSbPassStBkReclnUpwdDnwdSnsrHmPosLrnd_Val_read : Inport  Port=12
  IfVeSMSbPassStBlstOtwdInwdSnsrHmPosLrnd_Val_read : Inport  Port=13
  IfVeSMSbPassStCshnFrntUpwdDnwdSnsrHmPosLrnd_Val_read : Inport  Port=14
  IfVeSMSbPassStCshnRrUpwdDnwdSnsrHmPosLrnd_Val_read : Inport  Port=15
  IfVeSMSbPassStFrwdBkwdSnsrHmPosLrnd_Val_read : Inport  Port=16
  IfVeSMSbPassStFtUpwdDnwdSnsrHmPosLrnd_Val_read : Inport  Port=17
  IfVeSMSbPassStHdrstUpwdDnwdSnsrHmPosLrnd_Val_read : Inport  Port=18
  IfVeSMSbPassStLgrstUpwdDnwdSnsrHmPosLrnd_Val_read : Inport  Port=19
  IfVeSMSbSecRwLtStArmScrnSnsrHmPosLrnd_Val_read : Inport  Port=20
  IfVeSMSbSecRwLtStBkReclnUpwdDnwdSnsrHmPosLrnd_Val_read : Inport  Port=21
  IfVeSMSbSecRwLtStBlstOtwdInwdSnsrHmPosLrnd_Val_read : Inport  Port=22
  IfVeSMSbSecRwLtStCshnFrntUpwdDnwdSnsrHmPosLrnd_Val_read : Inport  Port=23
  IfVeSMSbSecRwLtStCshnRrUpwdDnwdSnsrHmPosLrnd_Val_read : Inport  Port=24
  IfVeSMSbSecRwLtStFrwdBkwdSnsrHmPosLrnd_Val_read : Inport  Port=25
  IfVeSMSbSecRwLtStLgrstUpwdDnwdSnsrHmPosLrnd_Val_read : Inport  Port=26
  IfVeSMSbSecRwLtStLtwdRtwdSnsrHmPosLrnd_Val_read : Inport  Port=27
  IfVeSMSbSecRwLtStHdrstUpwdDnwdSnsrHmPosLrnd_Val_read : Inport  Port=28
  IfVeSMSbSecRwRtStArmScrnSnsrHmPosLrnd_Val_read : Inport  Port=29
  IfVeSMSbSecRwRtStBkReclnUpwdDnwdSnsrHmPosLrnd_Val_read : Inport  Port=30
  IfVeSMSbSecRwRtStBlstOtwdInwdSnsrHmPosLrnd_Val_read : Inport  Port=31
  IfVeSMSbSecRwRtStCshnFrntUpwdDnwdSnsrHmPosLrnd_Val_read : Inport  Port=32
  IfVeSMSbSecRwRtStCshnRrUpwdDnwdSnsrHmPosLrnd_Val_read : Inport  Port=33
  IfVeSMSbSecRwRtStFrwdBkwdSnsrHmPosLrnd_Val_read : Inport  Port=34
  IfVeSMSbSecRwRtStLgrstUpwdDnwdSnsrHmPosLrnd_Val_read : Inport  Port=35
  IfVeSMSbSecRwRtStLtwdRtwdSnsrHmPosLrnd_Val_read : Inport  Port=36
  IfVeSMSbSecRwRtStHdrstUpwdDnwdSnsrHmPosLrnd_Val_read : Inport  Port=37
  IfVeSMSbThdRwLtStBkReclnUpwdDnwdSnsrHmPosLrnd_Val_read : Inport  Port=38
  IfVeSMSbThdRwLtStCshnFldUpwdDnwdSnsrHmPosLrnd_Val_read : Inport  Port=39
  IfVeSMSbThdRwLtStFrwdBkwdSnsrHmPosLrnd_Val_read : Inport  Port=40
  IfVeSMSbThdRwRtStBkReclnUpwdDnwdSnsrHmPosLrnd_Val_read : Inport  Port=41
  IfVeSMSbThdRwRtStCshnFldUpwdDnwdMovSnsrHmPosLrnd_Val_read : Inport  Port=42
  IfVeSMSbThdRwRtStFrwdBkwdSnsrHmPosLrnd_Val_read : Inport  Port=43
  IfVeSMSeStNumConfig_Val_read : Inport  Port=44
  IfVeSMSbPassStBkReclnUpwdDnwdMovConfig_Val_read : Inport  Port=45
  IfVeSMSbPassStFrwdBkwdMovConfig_Val_read : Inport  Port=46
  IfVeSMSbPassStFtUpwdDnwdMovConfig_Val_read : Inport  Port=47
  IfVeSMSbRrLtStFtUpwdDnwdSnsrHmPosLrnd_Val_read : Inport  Port=48
  IfVeSMSbRrRtStFtUpwdDnwdSnsrHmPosLrnd_Val_read : Inport  Port=49
  IfVeSMSbRrRtStFtUpwdMovConfig_Val_read : Inport  Port=50
  IfVeSMSbSecRwRtStBkReclnUpwdDnwdMovConfig_Val_read : Inport  Port=51
  IfVeSMSbSecRwRtStLgrstUpwdMovConfig_Val_read : Inport  Port=52
  IfVeSMSbSecRwRtStLtwdRtwdMovConfig_Val_read : Inport  Port=53
  IfVeSMSbSecRwRtStFrwdBkwdMovConfig_Val_read : Inport  Port=54
  IfVeSMSbSecRwRtStBlstOtwdInwdMovConfig_Val_read : Inport  Port=55
  IfVeSMSbSecRwRtStHdrstFrwdMovConfig_Val_read : Inport  Port=56
  IfVeSMSbSecRwRtStHdrstUpwdMovConfig_Val_read : Inport  Port=57
  IfVeSMSbSecRwRtStLgrstOtwdInwdMovConfig_Val_read : Inport  Port=58
  IfVeSMSbSecRwLtStHdrstFrwdBkwdSnsrHmPosLrnd_Val_read : Inport  Port=59
  IfVeSMSbSecRwLtStLgrstOtwdInwdSnsrHmPosLrnd_Val_read : Inport  Port=60
  IfVeSMSbSecRwRtStHdrstFrwdBkwdSnsrHmPosLrnd_Val_read : Inport  Port=61
  IfVeSMSbSecRwRtStLgrstOtwdInwdSnsrHmPosLrnd_Val_read : Inport  Port=62
  IfVeSMSbThdRwLtStBkReclnUpwdDnwdMovConfig_Val_read : Inport  Port=63
  IfVeSMSbThdRwLtStCshnFldUpwdDnwdMovConfig_Val_read : Inport  Port=64
  IfVeSMSbThdRwLtStFrwdBkwdMovConfig_Val_read : Inport  Port=65
  IfVeSMSbThdRwRtStBkReclnUpwdDnwdMovConfig_Val_read : Inport  Port=66
  IfVeSMSbThdRwRtStCshnFldUpwdDnwdMovConfig_Val_read : Inport  Port=67
  IfVeSMSbThdRwRtStFrwdBkwdMovConfig_Val_read : Inport  Port=68
  IfVeSMSbSecRwRtStArmScrnFrwdBkwdMovConfig_Val_read : Inport  Port=69
  IfVeSMSbSecRwRtStCshnFrntUpwdDnwdMovConfig_Val_read : Inport  Port=70
  IfVeSMSbPassStFldUpwdDnwdMovConfig_Val_read : Inport  Port=71
  IfVeSMSbPassStFldUpwdDnwdSnsrHmPosLrnd_Val_read : Inport  Port=72
  function : TriggerPort  TriggerType=function-call  VariantControl=(inherit)  SampleTimeType=periodic  SampleTime=-1
  DealPosLrndRunnable_sys : Subsystem
  PA_IfKeSMSbSeatMovBkRclnEnable_Val : Constant  Value=IfKeSMSbSeatMovBkRclnEnable_Val
  PA_IfKeSMSbSeatMovBlstOtwdInwdEnable_Val : Constant  Value=IfKeSMSbSeatMovBlstOtwdInwdEnable_Val
  PA_IfKeSMSbSeatMovCshnFldEnable_Val : Constant  Value=IfKeSMSbSeatMovCshnFldEnable_Val
  PA_IfKeSMSbSeatMovCushnFrtEnable_Val : Constant  Value=IfKeSMSbSeatMovCushnFrtEnable_Val
  PA_IfKeSMSbSeatMovFrwdBkwdEnable_Val : Constant  Value=IfKeSMSbSeatMovFrwdBkwdEnable_Val
  PA_IfKeSMSbSeatMovFtrstEnable_Val : Constant  Value=IfKeSMSbSeatMovFtrstEnable_Val
  PA_IfKeSMSbSeatMovLgrstEnable_Val : Constant  Value=IfKeSMSbSeatMovLgrstEnable_Val
  PA_IfKeSMSbSeatMovLtwdRtwdEnable_Val : Constant  Value=IfKeSMSbSeatMovLtwdRtwdEnable_Val
  PA_KeSMSbArmscreenMovEnable_Val : Constant  Value=KeSMSbArmscreenMovEnable_Val
  PA_KeSMSbIgnorePosLrnd_Val : Constant  Value=KeSMSbIgnorePosLrnd_Val
  PA_KeSMSbSeatMovHdFrwdBkwdEnable_Val : Constant  Value=KeSMSbSeatMovHdFrwdBkwdEnable_Val
  PA_KeSMSbSeatMovHdUpwdDnwdEnable_Val : Constant  Value=KeSMSbSeatMovHdUpwdDnwdEnable_Val
  PA_KeSMSbSeatMovLgrstExpdEnable_Val : Constant  Value=KeSMSbSeatMovLgrstExpdEnable_Val
  IfVeSMSbAcsEntryPosLrnd_Val_write : Outport
  IfVeSMSbDrvStPosLrnd_Val_write : Outport  Port=2
  IfVeSMSbFamilyLtPosLrnd_Val_write : Outport  Port=3
  IfVeSMSbFamilyRtPosLrnd_Val_write : Outport  Port=4
  IfVeSMSbIntimacyLPosLrnd_Val_write : Outport  Port=5
  IfVeSMSbIntimacyRPosLrnd_Val_write : Outport  Port=6
  IfVeSMSbLgrstCloseLtPosLrnd_Val_write : Outport  Port=7
  IfVeSMSbLgrstCloseRtPosLrnd_Val_write : Outport  Port=8
  IfVeSMSbLgrstOpenLtPosLrnd_Val_write : Outport  Port=9
  IfVeSMSbLgrstOpenRtPosLrnd_Val_write : Outport  Port=10
  IfVeSMSbLugLtPosLrnd_Val_write : Outport  Port=11
  IfVeSMSbLugRtPosLrnd_Val_write : Outport  Port=12
  IfVeSMSbLyingLtPosLrnd_Val_write : Outport  Port=13
  IfVeSMSbLyingRtPosLrnd_Val_write : Outport  Port=14
  IfVeSMSbAcsExitPosLrnd_Val_write : Outport  Port=15
  IfVeSMSbPassStPosLrnd_Val_write : Outport  Port=16
  IfVeSMSbVIPLtPosLrnd_Val_write : Outport  Port=17
  IfVeSMSbSecRwLtStPosLrnd_Val_write : Outport  Port=18
  IfVeSMSbVIPRtPosLrnd_Val_write : Outport  Port=19
  IfVeSMSbSecRwRtStPosLrnd_Val_write : Outport  Port=20
  IfVeSMSbRcvyLtPosLrnd_Val_write : Outport  Port=21
  IfVeSMSbThdRwLtStPosLrnd_Val_write : Outport  Port=22
  IfVeSMSbRcvyRtPosLrnd_Val_write : Outport  Port=23
  IfVeSMSbThdRwRtStPosLrnd_Val_write : Outport  Port=24
  IfVeSMSbAcsEntry4s2LPosLrnd_Val_write : Outport  Port=25
  IfVeSMSbAcsEntry4s2RPosLrnd_Val_write : Outport  Port=26
  IfVeSMSbAcsEntryAll4sBwdPosLrnd_Val_write : Outport  Port=27
  IfVeSMSbAcsEntryAll4sFwdPosLrnd_Val_write : Outport  Port=28
  IfVeSMSbAcsExit4s2LPosLrnd_Val_write : Outport  Port=29
  IfVeSMSbAcsExit4s2RPosLrnd_Val_write : Outport  Port=30
  IfVeSMSbPassReclinerPosLrnd_Val_write : Outport  Port=31
  IfVeSMSbunfold3LPosLrnd_Val_write : Outport  Port=32
  IfVeSMSbunfold3RPosLrnd_Val_write : Outport  Port=33
  IfVeSMSbVIPLtOutPosLrnd_Val_write : Outport  Port=34
  IfVeSMSbVIPRtOutPosLrnd_Val_write : Outport  Port=35
  IfVeSMSbWholeVehMemPosLrnd_Val_write : Outport  Port=36
  wires:
  DealPosLrndRunnable_sys/1(IfVeSMSbAcsEntryPosLrnd_Val_write) -> IfVeSMSbAcsEntryPosLrnd_Val_write/1
  DealPosLrndRunnable_sys/2(IfVeSMSbAcsExitPosLrnd_Val_write) -> IfVeSMSbAcsExitPosLrnd_Val_write/1
  DealPosLrndRunnable_sys/3(IfVeSMSbVIPLtPosLrnd_Val_write) -> IfVeSMSbVIPLtPosLrnd_Val_write/1
  DealPosLrndRunnable_sys/4(IfVeSMSbVIPRtPosLrnd_Val_write) -> IfVeSMSbVIPRtPosLrnd_Val_write/1
  DealPosLrndRunnable_sys/5(IfVeSMSbRcvyLtPosLrnd_Val_write) -> IfVeSMSbRcvyLtPosLrnd_Val_write/1
  DealPosLrndRunnable_sys/6(IfVeSMSbRcvyRtPosLrnd_Val_write) -> IfVeSMSbRcvyRtPosLrnd_Val_write/1
  DealPosLrndRunnable_sys/7(IfVeSMSbLugLtPosLrnd_Val_write) -> IfVeSMSbLugLtPosLrnd_Val_write/1
  DealPosLrndRunnable_sys/8(IfVeSMSbLugRtPosLrnd_Val_write) -> IfVeSMSbLugRtPosLrnd_Val_write/1
  DealPosLrndRunnable_sys/9(IfVeSMSbLyingLtPosLrnd) -> IfVeSMSbLyingLtPosLrnd_Val_write/1
  DealPosLrndRunnable_sys/10(IfVeSMSbLyingRtPosLrnd) -> IfVeSMSbLyingRtPosLrnd_Val_write/1
  DealPosLrndRunnable_sys/11(IfVeSMSbIntimacyLPosLrnd) -> IfVeSMSbIntimacyLPosLrnd_Val_write/1
  DealPosLrndRunnable_sys/12(IfVeSMSbFamilyLtPosLrnd) -> IfVeSMSbFamilyLtPosLrnd_Val_write/1
  DealPosLrndRunnable_sys/13(IfVeSMSbFamilyRtPosLrnd) -> IfVeSMSbFamilyRtPosLrnd_Val_write/1
  DealPosLrndRunnable_sys/14(IfVeSMSbDrvStPosLrnd_Val_write) -> IfVeSMSbDrvStPosLrnd_Val_write/1
  DealPosLrndRunnable_sys/15(IfVeSMSbPassStPosLrnd_Val_write) -> IfVeSMSbPassStPosLrnd_Val_write/1
  DealPosLrndRunnable_sys/16(IfVeSMSbSecRwLtStPosLrnd_Val_write) -> IfVeSMSbSecRwLtStPosLrnd_Val_write/1
  DealPosLrndRunnable_sys/17(IfVeSMSbSecRwRtStPosLrnd_Val_write) -> IfVeSMSbSecRwRtStPosLrnd_Val_write/1
  DealPosLrndRunnable_sys/18(IfVeSMSbThdRwLtStPosLrnd_Val_write) -> IfVeSMSbThdRwLtStPosLrnd_Val_write/1
  DealPosLrndRunnable_sys/19(IfVeSMSbThdRwRtStPosLrnd_Val_write) -> IfVeSMSbThdRwRtStPosLrnd_Val_write/1
  DealPosLrndRunnable_sys/20(IfVeSMSbLgrstOpenLtPosLrnd) -> IfVeSMSbLgrstOpenLtPosLrnd_Val_write/1
  DealPosLrndRunnable_sys/21(IfVeSMSbLgrstCloseLtPosLrnd) -> IfVeSMSbLgrstCloseLtPosLrnd_Val_write/1
  DealPosLrndRunnable_sys/22(IfVeSMSbLgrstOpenRtPosLrnd) -> IfVeSMSbLgrstOpenRtPosLrnd_Val_write/1
  DealPosLrndRunnable_sys/23(IfVeSMSbLgrstCloseRtPosLrnd) -> IfVeSMSbLgrstCloseRtPosLrnd_Val_write/1
  DealPosLrndRunnable_sys/24(IfVeSMSbIntimacyRPosLrnd) -> IfVeSMSbIntimacyRPosLrnd_Val_write/1
  IfVeSMSeStNumConfig_Val_read/1 -> DealPosLrndRunnable_sys/67(IfVeSMSeStNumConfig)
  PA_KeSMSbSeatMovHdFrwdBkwdEnable_Val/1 -> DealPosLrndRunnable_sys/74(KeSMSbSeatMovHdFrwdBkwdEnable)
  PA_KeSMSbSeatMovHdUpwdDnwdEnable_Val/1 -> DealPosLrndRunnable_sys/76(KeSMSbSeatMovHdUpwdDnwdEnable)
  PA_KeSMSbSeatMovLgrstExpdEnable_Val/1 -> DealPosLrndRunnable_sys/75(KeSMSbSeatMovLgrstExpdEnable)
  IfVeSMSbDrvStBkReclnUpwdDnwdMovConfig_Val_read/1 -> DealPosLrndRunnable_sys/51(DrvStBkReclnUpwdDnwdMovConfig)
  IfVeSMSbDrvStFrwdBkwdMovConfig_Val_read/1 -> DealPosLrndRunnable_sys/52(DrvStFrwdBkwdMovConfig)
  IfVeSMSbDrvStFtUpwdDnwdMovConfig_Val_read/1 -> DealPosLrndRunnable_sys/53(DrvStFtUpwdDnwdMovConfig)
  PA_KeSMSbIgnorePosLrnd_Val/1 -> DealPosLrndRunnable_sys/49(KeSMSbIgnorePosLrnd)
  PA_IfKeSMSbSeatMovLgrstEnable_Val/1 -> DealPosLrndRunnable_sys/47(KeSMSbSeatMovLgrstEnable)
  PA_IfKeSMSbSeatMovLtwdRtwdEnable_Val/1 -> DealPosLrndRunnable_sys/48(KeSMSbSeatMovLtwdRtwdEnable)
  PA_KeSMSbArmscreenMovEnable_Val/1 -> DealPosLrndRunnable_sys/50(KeSMSbArmscreenMovEnable)
  PA_IfKeSMSbSeatMovFtrstEnable_Val/1 -> DealPosLrndRunnable_sys/46(KeSMSbSeatMovFtrstEnable)
  PA_IfKeSMSbSeatMovFrwdBkwdEnable_Val/1 -> DealPosLrndRunnable_sys/45(KeSMSbSeatMovFrwdBkwdEnable)
  PA_IfKeSMSbSeatMovCshnFldEnable_Val/1 -> DealPosLrndRunnable_sys/44(KeSMSbSeatMovCshnFldEnable)
  PA_IfKeSMSbSeatMovBlstOtwdInwdEnable_Val/1 -> DealPosLrndRunnable_sys/43(KeSMSbSeatMovBlstOtwdInwdEnable)
  PA_IfKeSMSbSeatMovBkRclnEnable_Val/1 -> DealPosLrndRunnable_sys/42(KeSMSbSeatMovBkRclnEnable)
  IfVeSMSbDrvStBkReclnUpwdDnwdSnsrHmPosLrnd_Val_read/1 -> DealPosLrndRunnable_sys/1(DrvStBkReclnUpwdDnwdSnsrHmPosLrnd)
  IfVeSMSbDrvStBlstOtwdInwdSnsrHmPosLrnd_Val_read/1 -> DealPosLrndRunnable_sys/2(IfVeSMSbDrvStBlstOtwdInwdSnsrHmPosLrnd_Val_read)
  IfVeSMSbDrvStCshnFrntUpwdDnwdSnsrHmPosLrnd_Val_read/1 -> DealPosLrndRunnable_sys/3(IfVeSMSbDrvStCshnFrntUpwdDnwdSnsrHmPosLrnd_Val_read)
  IfVeSMSbDrvStCshnRrUpwdDnwdSnsrHmPosLrnd_Val_read/1 -> DealPosLrndRunnable_sys/4(IfVeSMSbDrvStCshnRrUpwdDnwdSnsrHmPosLrnd_Val_read)
  IfVeSMSbDrvStFrwdBkwdSnsrHmPosLrnd_Val_read/1 -> DealPosLrndRunnable_sys/5(DrvStFrwdBkwdSnsrHmPosLrnd)
  IfVeSMSbDrvStFtUpwdDnwdSnsrHmPosLrnd_Val_read/1 -> DealPosLrndRunnable_sys/6(DrvStFtUpwdDnwdSnsrHmPosLrnd)
  IfVeSMSbDrvStHdrstUpwdDnwdSnsrHmPosLrnd_Val_read/1 -> DealPosLrndRunnable_sys/7(IfVeSMSbDrvStHdrstUpwdDnwdSnsrHmPosLrnd_Val_read)
  IfVeSMSbDrvStLgrstUpwdDnwdSnsrHmPosLrnd_Val_read/1 -> DealPosLrndRunnable_sys/8(IfVeSMSbDrvStLgrstUpwdDnwdSnsrHmPosLrnd_Val_read)
  IfVeSMSbPassStBkReclnUpwdDnwdMovConfig_Val_read/1 -> DealPosLrndRunnable_sys/54(PassStBkReclnUpwdDnwdMovConfig)
  IfVeSMSbPassStFrwdBkwdMovConfig_Val_read/1 -> DealPosLrndRunnable_sys/55(PassStFrwdBkwdMovConfig)
  IfVeSMSbPassStFtUpwdDnwdMovConfig_Val_read/1 -> DealPosLrndRunnable_sys/56(PassStFtUpwdDnwdMovConfig)
  IfVeSMSbPassStBkReclnUpwdDnwdSnsrHmPosLrnd_Val_read/1 -> DealPosLrndRunnable_sys/9(PassStBkReclnUpwdDnwdSnsrHmPosLrnd)
  IfVeSMSbPassStBlstOtwdInwdSnsrHmPosLrnd_Val_read/1 -> DealPosLrndRunnable_sys/10(IfVeSMSbPassStBlstOtwdInwdSnsrHmPosLrnd_Val_read)
  IfVeSMSbPassStCshnFrntUpwdDnwdSnsrHmPosLrnd_Val_read/1 -> DealPosLrndRunnable_sys/11(IfVeSMSbPassStCshnFrntUpwdDnwdSnsrHmPosLrnd_Val_read)
  IfVeSMSbPassStCshnRrUpwdDnwdSnsrHmPosLrnd_Val_read/1 -> DealPosLrndRunnable_sys/12(IfVeSMSbPassStCshnRrUpwdDnwdSnsrHmPosLrnd_Val_read)
  IfVeSMSbPassStFrwdBkwdSnsrHmPosLrnd_Val_read/1 -> DealPosLrndRunnable_sys/13(PassStFrwdBkwdSnsrHmPosLrnd)
  IfVeSMSbPassStFtUpwdDnwdSnsrHmPosLrnd_Val_read/1 -> DealPosLrndRunnable_sys/14(PassStFtUpwdDnwdSnsrHmPosLrnd)
  IfVeSMSbPassStHdrstUpwdDnwdSnsrHmPosLrnd_Val_read/1 -> DealPosLrndRunnable_sys/15(IfVeSMSbPassStHdrstUpwdDnwdSnsrHmPosLrnd_Val_read)
  IfVeSMSbPassStLgrstUpwdDnwdSnsrHmPosLrnd_Val_read/1 -> DealPosLrndRunnable_sys/16(IfVeSMSbPassStLgrstUpwdDnwdSnsrHmPosLrnd_Val_read)
  IfVeSMSbRrLtStFtUpwdDnwdSnsrHmPosLrnd_Val_read/1 -> DealPosLrndRunnable_sys/68(RrLtStFtUpwdDnwdSnsrHmPosLrnd)
  IfVeSMSbRrRtStFtUpwdDnwdSnsrHmPosLrnd_Val_read/1 -> DealPosLrndRunnable_sys/71(RrRtStFtUpwdDnwdSnsrHmPosLrnd)
  IfVeSMSbRrRtStFtUpwdMovConfig_Val_read/1 -> DealPosLrndRunnable_sys/77(IfVeSMSbRrRtStFtUpwdMovConfig)
  IfVeSMSbSecRwRtStFrwdBkwdMovConfig_Val_read/1 -> DealPosLrndRunnable_sys/58(SecRwRtStFrwdBkwdMovConfig)
  IfVeSMSbSecRwRtStLtwdRtwdMovConfig_Val_read/1 -> DealPosLrndRunnable_sys/59(SecRwRtStLtwdRtwdMovConfig)
  IfVeSMSbSecRwRtStBkReclnUpwdDnwdMovConfig_Val_read/1 -> DealPosLrndRunnable_sys/57(SecRwRtStBkReclnUpwdDnwdMovConfig)
  IfVeSMSbSecRwRtStLgrstUpwdMovConfig_Val_read/1 -> DealPosLrndRunnable_sys/60(SecRwRtStLgrstUpwdMovConfig)
  IfVeSMSbSecRwRtStHdrstFrwdMovConfig_Val_read/1 -> DealPosLrndRunnable_sys/78(IfVeSMSbSecRwRtStHdrstFrwdMovConfig)
  IfVeSMSbSecRwRtStLgrstOtwdInwdMovConfig_Val_read/1 -> DealPosLrndRunnable_sys/79(IfVeSMSbSecRwRtStLgrstOtwdInwdMovConfig)
  IfVeSMSbSecRwRtStHdrstUpwdMovConfig_Val_read/1 -> DealPosLrndRunnable_sys/80(IfVeSMSbSecRwRtStHdrstUpwdMovConfig)
  IfVeSMSbSecRwRtStBlstOtwdInwdMovConfig_Val_read/1 -> DealPosLrndRunnable_sys/19(SecRwRtStBlstOtwdInwdMovConfig)
  IfVeSMSbSecRwLtStArmScrnSnsrHmPosLrnd_Val_read/1 -> DealPosLrndRunnable_sys/17(SecRwLtStArmScrnSnsrHmPosLrnd)
  IfVeSMSbSecRwLtStBkReclnUpwdDnwdSnsrHmPosLrnd_Val_read/1 -> DealPosLrndRunnable_sys/18(SecRwLtStBkReclnUpwdDnwdSnsrHmPosLrnd)
  IfVeSMSbSecRwLtStBlstOtwdInwdSnsrHmPosLrnd_Val_read/1 -> DealPosLrndRunnable_sys/20(IfVeSMSbSecRwLtStBlstOtwdInwdSnsrHmPosLrnd_Val_read)
  IfVeSMSbSecRwLtStCshnFrntUpwdDnwdSnsrHmPosLrnd_Val_read/1 -> DealPosLrndRunnable_sys/21(IfVeSMSbSecRwLtStCshnFrntUpwdDnwdSnsrHmPosLrnd_Val_read)
  IfVeSMSbSecRwLtStCshnRrUpwdDnwdSnsrHmPosLrnd_Val_read/1 -> DealPosLrndRunnable_sys/22(IfVeSMSbSecRwLtStCshnRrUpwdDnwdSnsrHmPosLrnd_Val_read)
  IfVeSMSbSecRwLtStFrwdBkwdSnsrHmPosLrnd_Val_read/1 -> DealPosLrndRunnable_sys/23(SecRwLtStFrwdBkwdSnsrHmPosLrnd)
  IfVeSMSbSecRwLtStLgrstUpwdDnwdSnsrHmPosLrnd_Val_read/1 -> DealPosLrndRunnable_sys/24(SecRwLtStLgrstUpwdDnwdSnsrHmPosLrnd)
  IfVeSMSbSecRwLtStLtwdRtwdSnsrHmPosLrnd_Val_read/1 -> DealPosLrndRunnable_sys/25(SecRwLtStLtwdRtwdSnsrHmPosLrnd)
  IfVeSMSbSecRwLtStHdrstUpwdDnwdSnsrHmPosLrnd_Val_read/1 -> DealPosLrndRunnable_sys/26(IfVeSMSbSecRwLtStHdrstUpwdDnwdSnsrHmPosLrnd_Val_read)
  IfVeSMSbSecRwRtStArmScrnSnsrHmPosLrnd_Val_read/1 -> DealPosLrndRunnable_sys/27(IfVeSMSbSecRwRtStArmScrnSnsrHmPosLrnd_Val_read)
  IfVeSMSbSecRwLtStHdrstFrwdBkwdSnsrHmPosLrnd_Val_read/1 -> DealPosLrndRunnable_sys/69(SecRwLtStHdrstFrwdBkwdSnsrHmPosLrnd)
  IfVeSMSbSecRwLtStLgrstOtwdInwdSnsrHmPosLrnd_Val_read/1 -> DealPosLrndRunnable_sys/70(SecRwLtStLgrstOtwdInwdSnsrHmPosLrnd)
  IfVeSMSbSecRwRtStBkReclnUpwdDnwdSnsrHmPosLrnd_Val_read/1 -> DealPosLrndRunnable_sys/28(SecRwRtStBkReclnUpwdDnwdSnsrHmPosLrnd)
  IfVeSMSbSecRwRtStBlstOtwdInwdSnsrHmPosLrnd_Val_read/1 -> DealPosLrndRunnable_sys/29(IfVeSMSbSecRwRtStBlstOtwdInwdSnsrHmPosLrnd_Val_read)
  IfVeSMSbSecRwRtStCshnFrntUpwdDnwdSnsrHmPosLrnd_Val_read/1 -> DealPosLrndRunnable_sys/30(IfVeSMSbSecRwRtStCshnFrntUpwdDnwdSnsrHmPosLrnd_Val_read)
  IfVeSMSbSecRwRtStCshnRrUpwdDnwdSnsrHmPosLrnd_Val_read/1 -> DealPosLrndRunnable_sys/31(IfVeSMSbSecRwRtStCshnRrUpwdDnwdSnsrHmPosLrnd_Val_read)
  IfVeSMSbSecRwRtStFrwdBkwdSnsrHmPosLrnd_Val_read/1 -> DealPosLrndRunnable_sys/32(SecRwRtStFrwdBkwdSnsrHmPosLrnd)
  IfVeSMSbSecRwRtStLgrstUpwdDnwdSnsrHmPosLrnd_Val_read/1 -> DealPosLrndRunnable_sys/33(SecRwRtStLgrstUpwdDnwdSnsrHmPosLrnd)
  IfVeSMSbSecRwRtStLtwdRtwdSnsrHmPosLrnd_Val_read/1 -> DealPosLrndRunnable_sys/34(SecRwRtStLtwdRtwdSnsrHmPosLrnd)
  IfVeSMSbSecRwRtStHdrstUpwdDnwdSnsrHmPosLrnd_Val_read/1 -> DealPosLrndRunnable_sys/35(IfVeSMSbSecRwRtStHdrstUpwdDnwdSnsrHmPosLrnd_Val_read)
  IfVeSMSbSecRwRtStHdrstFrwdBkwdSnsrHmPosLrnd_Val_read/1 -> DealPosLrndRunnable_sys/72(SecRwRtStHdrstFrwdBkwdSnsrHmPosLrnd)
  IfVeSMSbSecRwRtStLgrstOtwdInwdSnsrHmPosLrnd_Val_read/1 -> DealPosLrndRunnable_sys/73(SecRwRtStLgrstOtwdInwdSnsrHmPosLrnd)
  IfVeSMSbThdRwLtStBkReclnUpwdDnwdMovConfig_Val_read/1 -> DealPosLrndRunnable_sys/61(ThdRwLtStBkReclnUpwdDnwdMovConfig)
  IfVeSMSbThdRwLtStCshnFldUpwdDnwdMovConfig_Val_read/1 -> DealPosLrndRunnable_sys/62(ThdRwLtStCshnFldUpwdDnwdMovConfig)
  IfVeSMSbThdRwRtStFrwdBkwdMovConfig_Val_read/1 -> DealPosLrndRunnable_sys/66(ThdRwRtStFrwdBkwdMovConfig)
  IfVeSMSbThdRwLtStFrwdBkwdMovConfig_Val_read/1 -> DealPosLrndRunnable_sys/63(ThdRwLtStFrwdBkwdMovConfig)
  IfVeSMSbThdRwRtStBkReclnUpwdDnwdMovConfig_Val_read/1 -> DealPosLrndRunnable_sys/64(ThdRwRtStBkReclnUpwdDnwdMovConfig)
  IfVeSMSbThdRwRtStCshnFldUpwdDnwdMovConfig_Val_read/1 -> DealPosLrndRunnable_sys/65(ThdRwRtStCshnFldUpwdDnwdMovConfig)
  IfVeSMSbThdRwLtStBkReclnUpwdDnwdSnsrHmPosLrnd_Val_read/1 -> DealPosLrndRunnable_sys/36(ThdRwLtStBkReclnUpwdDnwdSnsrHmPosLrnd)
  IfVeSMSbThdRwLtStCshnFldUpwdDnwdSnsrHmPosLrnd_Val_read/1 -> DealPosLrndRunnable_sys/37(ThdRwLtStCshnFldUpwdDnwdSnsrHmPosLrnd)
  IfVeSMSbThdRwLtStFrwdBkwdSnsrHmPosLrnd_Val_read/1 -> DealPosLrndRunnable_sys/38(ThdRwLtStFrwdBkwdSnsrHmPosLrnd)
  IfVeSMSbThdRwRtStBkReclnUpwdDnwdSnsrHmPosLrnd_Val_read/1 -> DealPosLrndRunnable_sys/39(ThdRwRtStBkReclnUpwdDnwdSnsrHmPosLrnd)
  IfVeSMSbThdRwRtStCshnFldUpwdDnwdMovSnsrHmPosLrnd_Val_read/1 -> DealPosLrndRunnable_sys/40(ThdRwRtStCshnFldUpwdDnwdSnsrHmPosLrnd)
  IfVeSMSbThdRwRtStFrwdBkwdSnsrHmPosLrnd_Val_read/1 -> DealPosLrndRunnable_sys/41(ThdRwRtStFrwdBkwdSnsrHmPosLrnd)
  DealPosLrndRunnable_sys/25(IfVeSMSbAcsEntry4s2LPosLrnd) -> IfVeSMSbAcsEntry4s2LPosLrnd_Val_write/1
  DealPosLrndRunnable_sys/26(IfVeSMSbAcsEntry4s2RPosLrnd) -> IfVeSMSbAcsEntry4s2RPosLrnd_Val_write/1
  DealPosLrndRunnable_sys/27(IfVeSMSbAcsExit4s2LPosLrnd) -> IfVeSMSbAcsExit4s2LPosLrnd_Val_write/1
  DealPosLrndRunnable_sys/28(IfVeSMSbAcsExit4s2RPosLrnd) -> IfVeSMSbAcsExit4s2RPosLrnd_Val_write/1
  DealPosLrndRunnable_sys/29(IfVeSMSbAcsEntryAll4sBwdPosLrnd) -> IfVeSMSbAcsEntryAll4sBwdPosLrnd_Val_write/1
  DealPosLrndRunnable_sys/30(IfVeSMSbAcsEntryAll4sFwdPosLrnd) -> IfVeSMSbAcsEntryAll4sFwdPosLrnd_Val_write/1
  IfVeSMSbSecRwRtStArmScrnFrwdBkwdMovConfig_Val_read/1 -> DealPosLrndRunnable_sys/81(IfVeSMSbSecRwRtStArmScrnFrwdBkwdMovConfig)
  IfVeSMSbSecRwRtStCshnFrntUpwdDnwdMovConfig_Val_read/1 -> DealPosLrndRunnable_sys/82("IfVeSMSbSecRwRtStCshnFrntUpwdDnwdMovConfig ")
  PA_IfKeSMSbSeatMovCushnFrtEnable_Val/1 -> DealPosLrndRunnable_sys/83(IfKeSMSbSeatMovCushnFrtEnable)
  IfVeSMSbPassStFldUpwdDnwdMovConfig_Val_read/1 -> DealPosLrndRunnable_sys/84(IfVeSMSbPassStFldUpwdDnwdMovConfig)
  IfVeSMSbPassStFldUpwdDnwdSnsrHmPosLrnd_Val_read/1 -> DealPosLrndRunnable_sys/85(IfVeSMSbPassStFldUpwdDnwdSnsrHmPosLrnd_Val_read)
  DealPosLrndRunnable_sys/31(IfVeSMSbPassReclinerPosLrnd_Val_write) -> IfVeSMSbPassReclinerPosLrnd_Val_write/1
  DealPosLrndRunnable_sys/32(IfVeSMSbunfold3LPosLrnd_Val_write) -> IfVeSMSbunfold3LPosLrnd_Val_write/1
  DealPosLrndRunnable_sys/33(IfVeSMSbunfold3RPosLrnd_Val_write) -> IfVeSMSbunfold3RPosLrnd_Val_write/1
  DealPosLrndRunnable_sys/34(IfVeSMSbVIPLtOutPosLrnd_Val_write) -> IfVeSMSbVIPLtOutPosLrnd_Val_write/1
  DealPosLrndRunnable_sys/35(IfVeSMSbVIPRtOutPosLrnd_Val_write) -> IfVeSMSbVIPRtOutPosLrnd_Val_write/1
  DealPosLrndRunnable_sys/36(IfVeSMSbWholeVehMemPosLrnd_Val_write) -> IfVeSMSbWholeVehMemPosLrnd_Val_write/1

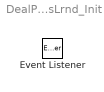
== system DealPosLrnd/DealPosLrnd_Init ==
  Event Listener : EventListener  EventName=reset
